simulink model "Cyclo_converter"  (R2021a)
settings: Solver=VariableStepAuto  StartTime=0.0  StopTime=0.15  FixedStep=0.01  RelTol=1e-3
libraries: spsThyristorLib x8, spsIdealSwitchLib x2, spsVoltageMeasurementLib x2, spsACVoltageSourceLib x1, spsSeriesRLCBranchLib x1, spspowerguiLib x1
settings Model: Creator=Davie  LastModifiedBy=Davie

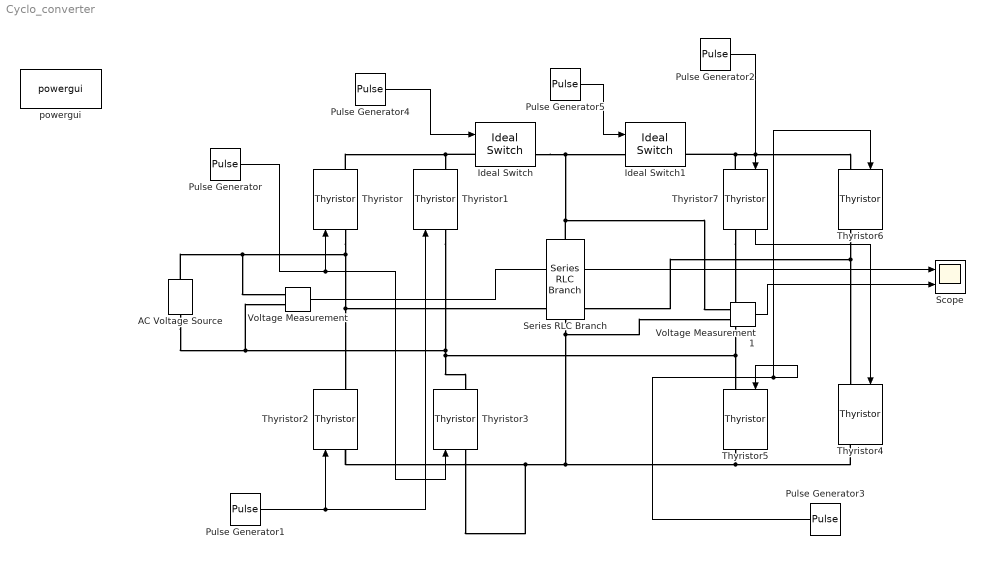
== system Cyclo_converter ==
  AC Voltage Source : spsACVoltageSourceLib/AC Voltage Source  Amplitude=100  Phase=0  Frequency=50  SampleTime=0  Measurements=None  BusType=swing  Pref=10e3  Qref=0  Qmin=-inf  Qmax=+inf
  Ideal Switch : spsIdealSwitchLib/Ideal Switch  Ron=0.001  Lon=0  IC=0  Rs=1e5  Cs=inf  Measurements=on
  Ideal Switch1 : spsIdealSwitchLib/Ideal Switch  Ron=0.001  Lon=0  IC=0  Rs=1e5  Cs=inf  Measurements=on
  Pulse Generator : DiscretePulseGenerator  PulseType=Time based  Period=0.02  PulseWidth=50  PhaseDelay=(30/360)*0.002
  Pulse Generator1 : DiscretePulseGenerator  PulseType=Time based  Period=0.02  PulseWidth=50  PhaseDelay=(210/360)*0.002
  Pulse Generator2 : DiscretePulseGenerator  PulseType=Time based  Period=0.02  PulseWidth=50  PhaseDelay=(30/360)*0.002
  Pulse Generator3 : DiscretePulseGenerator  PulseType=Time based  Period=0.02  PulseWidth=50  PhaseDelay=(210/360)*0.002
  Pulse Generator4 : DiscretePulseGenerator  PulseType=Time based  Period=0.08  PulseWidth=50
  Pulse Generator5 : DiscretePulseGenerator  PulseType=Time based  Period=0.08  PulseWidth=50  PhaseDelay=0.04
  Scope : Scope  NumInputPorts=2
  Series RLC Branch : spsSeriesRLCBranchLib/Series RLC Branch  LConnTagsString=__new0  RConnTagsString=__new0  BranchType=R  Resistance=1  Inductance=1e-3  SetiL0=off  InitialCurrent=0  Capacitance=1e-6  Setx0=off  InitialVoltage=0  Measurements=None
  Thyristor{,1..7} (8 alike) : spsThyristorLib/Thyristor  Ron=0.001  Lon=0  Vf=0.8  IC=0  Rs=500  Cs=250e-9  Measurements=on
  Voltage Measurement : spsVoltageMeasurementLib/Voltage Measurement  PhasorSimulation=off  OutputType=Complex  PSBequivalent=0
  Voltage Measurement1 : spsVoltageMeasurementLib/Voltage Measurement  PhasorSimulation=off  OutputType=Complex  PSBequivalent=0
  powergui : spspowerguiLib/powergui  Priority=1  SimulationMode=Discrete  SampleTime=0.05e-6  frequency=60  Iterations=50  frequencyindice=50  Pbase=100e6  ErrMax=1e-4  UnitsV=kV  UnitsW=MW  buscounter=0  FunctionMessages=off  echomessages=off  EnableUseOfTLC=off  CurrentSourceSwitches=off  DisableSnubberDevices=off  DisableRonSwitches=off  DisableVfSwitches=off  DisplayEquations=off  AutomaticDiscreteSolvers=off  SolverType=Tustin/Backward Euler (TBE)  Interpol=off  ExternalGateDelay=off  methode=off  Ts=100  x0status=blocks  SPID=on  SwTol=0  HookPort=off  NonlinearTolerance=1e-4  nMaxIteration=100  ContinueOnMaxIteration=off  RestoreLinks=warning  ResistiveCurrentMeasurement=off  Frange=[0:2:500]  Ylog=off  Xlog=on  ShowGrid=off  save=off  variable=ZData  structure=0  ZoomFFT=off  StartTime=0.0  cycles=1  DisplayStyle=1  fundamental=60  FreqAxis=off  MaxFrequency=1000  frequencyindicesteady=1  RmsSteady=1  display=off
  wires:
  Pulse Generator/1 -> Thyristor3/1, Thyristor/1
  Pulse Generator1/1 -> Thyristor1/1, Thyristor2/1
  Pulse Generator3/1 -> Thyristor6/1, Thyristor5/1
  Pulse Generator2/1 -> Thyristor4/1, Thyristor7/1
  Voltage Measurement/1 -> Scope/1
  Voltage Measurement1/1 -> Scope/2
  Pulse Generator4/1 -> Ideal Switch/1
  Pulse Generator5/1 -> Ideal Switch1/1
  connections:
  Thyristor/RConn1 -- Ideal Switch/LConn1 -- Thyristor1/RConn1
  Thyristor2/LConn1 -- Thyristor3/LConn1 -- Series RLC Branch/RConn1 -- Voltage Measurement1/LConn2 -- Thyristor5/RConn1 -- Thyristor4/RConn1
  Thyristor1/LConn1 -- Thyristor7/RConn1 -- Thyristor5/LConn1 -- Thyristor3/RConn1 -- AC Voltage Source/LConn1 -- Voltage Measurement/LConn2
  Thyristor/LConn1 -- Thyristor2/RConn1 -- Thyristor4/LConn1 -- Thyristor6/RConn1 -- AC Voltage Source/RConn1 -- Voltage Measurement/LConn1
  Series RLC Branch/LConn1 -- Ideal Switch1/LConn1 -- Ideal Switch/RConn1 -- Voltage Measurement1/LConn1
  Thyristor7/LConn1 -- Ideal Switch1/RConn1 -- Thyristor6/LConn1
